simulink model "PI_controller"  (R2022b)
settings: Solver=VariableStepAuto  StartTime=0.0  StopTime=10.0  RelTol=1e-3
settings Model: Creator=yasso  LastModifiedBy=yasso

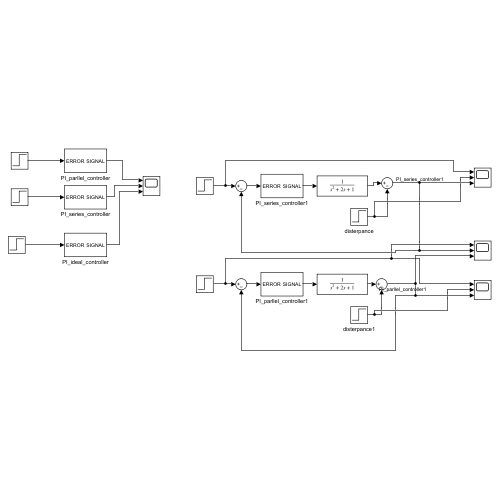
[thumbnail: Simulink's stored preview of the top-level diagram]
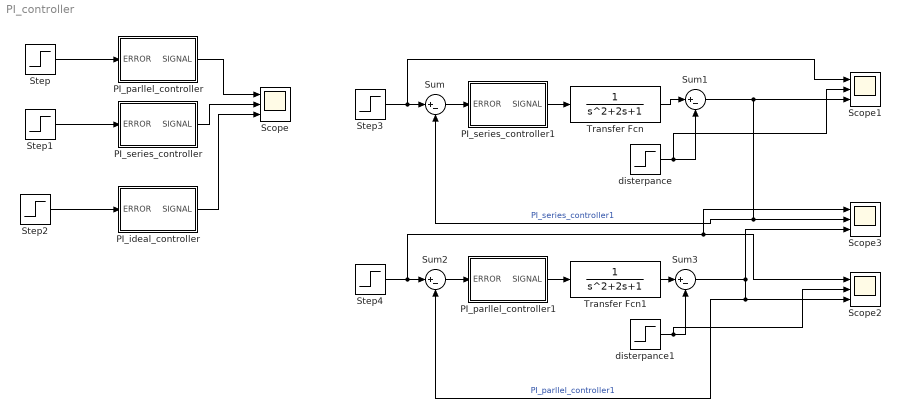
== system PI_controller ==
  PI_ideal_controller : Subsystem
  PI_parllel_controller : Subsystem
  PI_parllel_controller1 : Subsystem
  PI_series_controller : Subsystem
  PI_series_controller1 : Subsystem
  Scope{,1..3} (4 alike) : Scope  NumInputPorts=3
  Step{,1..4} (5 alike) : Step  SampleTime=0
  Sum{,1..3} (4 alike) : Sum  Inputs=|+-
  Transfer Fcn : TransferFcn
  Transfer Fcn1 : TransferFcn
  disterpance : Step  Time=4  After=0.4  SampleTime=0
  disterpance1 : Step  Time=4  After=0.4  SampleTime=0
  wires:
  Step/1 -> PI_parllel_controller/1(ERROR)
  PI_parllel_controller/1(SIGNAL) -> Scope/1
  PI_series_controller/1(SIGNAL) -> Scope/2
  Step1/1 -> PI_series_controller/1(ERROR)
  Step2/1 -> PI_ideal_controller/1(ERROR)
  PI_ideal_controller/1(SIGNAL) -> Scope/3
  Step3/1 -> Scope1/1, Sum/1
  Sum/1 -> PI_series_controller1/1(ERROR)
  PI_series_controller1/1(SIGNAL) -> Transfer Fcn/1
  Transfer Fcn/1 -> Sum1/1
  disterpance/1 -> Scope1/2, Sum1/2
  disterpance1/1 -> Sum3/2, Scope2/2
  Sum3/1 -> Scope3/3, Sum2/2, Scope2/3  "PI_parllel_controller1"
  Transfer Fcn1/1 -> Sum3/1
  PI_parllel_controller1/1(SIGNAL) -> Transfer Fcn1/1
  Sum2/1 -> PI_parllel_controller1/1(ERROR)
  Step4/1 -> Sum2/1, Scope2/1, Scope3/1
  Sum1/1 -> Sum/2, Scope3/2, Scope1/3  "PI_series_controller1"

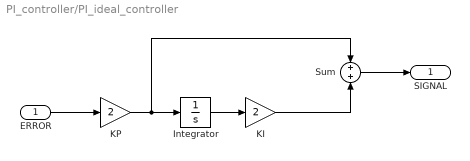
== system PI_controller/PI_ideal_controller ==
  ERROR : Inport
  Integrator : Integrator
  KI : Gain  Gain=2
  KP : Gain  Gain=2
  Sum : Sum  Inputs=+|+
  SIGNAL : Outport
  wires:
  KP/1 -> Integrator/1, Sum/1
  KI/1 -> Sum/2
  ERROR/1 -> KP/1
  Integrator/1 -> KI/1
  Sum/1 -> SIGNAL/1

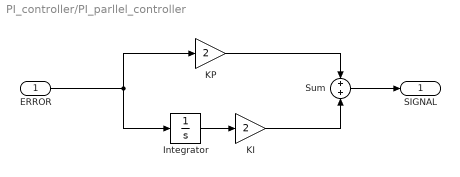
== system PI_controller/PI_parllel_controller ==
  ERROR : Inport
  Integrator : Integrator
  KI : Gain  Gain=2
  KP : Gain  Gain=2
  Sum : Sum  Inputs=+|+
  SIGNAL : Outport
  wires:
  KI/1 -> Sum/2
  ERROR/1 -> KP/1, Integrator/1
  KP/1 -> Sum/1
  Integrator/1 -> KI/1
  Sum/1 -> SIGNAL/1

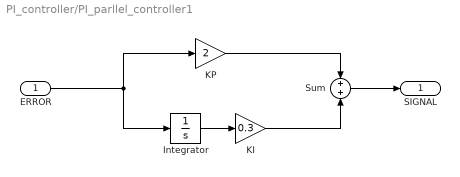
== system PI_controller/PI_parllel_controller1 ==
  ERROR : Inport
  Integrator : Integrator
  KI : Gain  Gain=0.3
  KP : Gain  Gain=2
  Sum : Sum  Inputs=+|+
  SIGNAL : Outport
  wires:
  Sum/1 -> SIGNAL/1
  Integrator/1 -> KI/1
  KP/1 -> Sum/1
  ERROR/1 -> Integrator/1, KP/1
  KI/1 -> Sum/2

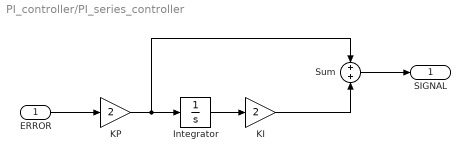
== system PI_controller/PI_series_controller ==
  ERROR : Inport
  Integrator : Integrator
  KI : Gain  Gain=2
  KP : Gain  Gain=2
  Sum : Sum  Inputs=+|+
  SIGNAL : Outport
  wires:
  Sum/1 -> SIGNAL/1
  Integrator/1 -> KI/1
  ERROR/1 -> KP/1
  KI/1 -> Sum/2
  KP/1 -> Sum/1, Integrator/1

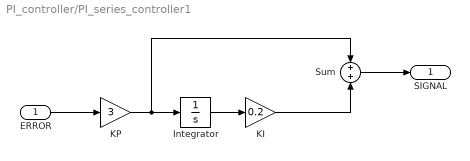
== system PI_controller/PI_series_controller1 ==
  ERROR : Inport
  Integrator : Integrator
  KI : Gain  Gain=0.2
  KP : Gain  Gain=3
  Sum : Sum  Inputs=+|+
  SIGNAL : Outport
  wires:
  KP/1 -> Integrator/1, Sum/1
  KI/1 -> Sum/2
  ERROR/1 -> KP/1
  Integrator/1 -> KI/1
  Sum/1 -> SIGNAL/1
